simulink model "Stateflow_SD104"  (R2015b)
settings: Solver=FixedStepAuto  StartTime=0.0  StopTime=20  RelTol=1e-3
settings Model: Creator=amyyang  LastModifiedBy=amyyang
settings OptimizationCC: DefaultParameterBehavior=Inlined  OptimizeModelRefInitCode=on  LifeSpan=1
settings RTWCC: SystemTargetFile=ert.tlc  GenCodeOnly=on  TemplateMakefile=ert_default_tmf  Description=Embedded Coder  GenerateReport=on  IncludeHyperlinkInReport=on  LaunchReport=on  GenerateTraceInfo=on  GenerateTraceReport=on  GenerateTraceReportSl=on  GenerateTraceReportSf=on  GenerateTraceReportEml=on
settings CodeAppCC: IgnoreCustomStorageClasses=off
settings ERTTargetCC: GenerateSampleERTMain=on  InlinedParameterPlacement=NonHierarchical  ERTCustomFileTemplate=example_file_process.tlc

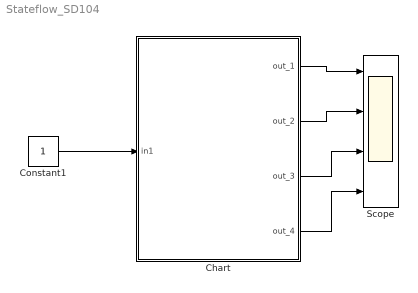
== system Stateflow_SD104 ==
  Chart : Stateflow chart  TreatAsAtomicUnit=on
  Constant1 : Constant
  Scope : Scope  NumInputPorts=4
  wires:
  Constant1/1 -> Chart/1(in1)
  Chart/1(out_1) -> Scope/1
  Chart/2(out_2) -> Scope/2
  Chart/3(out_3) -> Scope/3
  Chart/4(out_4) -> Scope/4

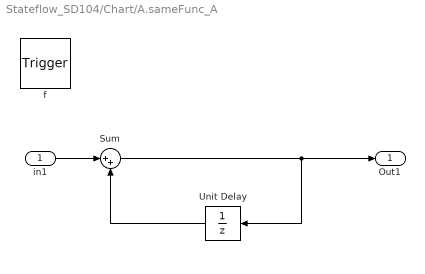
== system Stateflow_SD104/Chart/A.sameFunc_A ==
  in1 : Inport  OutDataTypeStr=double  PortDimensions=1
  f : TriggerPort  TriggerType=function-call
      settings: CopyFcn=Stateflow.SLINSF.SimulinkMan.removeBlockPreDeleteFcn  PreDeleteFcn=Stateflow.SLINSF.SimulinkMan.unsafePredeleteFcn
  Sum : Sum  Inputs=|++
  Unit Delay : UnitDelay  SampleTime=-1
  Out1 : Outport
  wires:
  in1/1 -> Sum/1
  Sum/1 -> Unit Delay/1, Out1/1
  Unit Delay/1 -> Sum/2

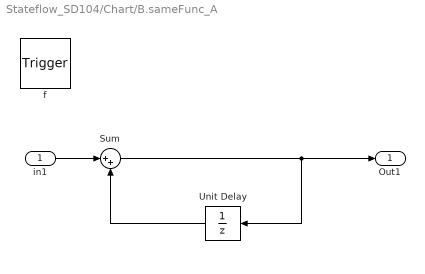
== system Stateflow_SD104/Chart/B.sameFunc_A ==
  in1 : Inport  OutDataTypeStr=double  PortDimensions=1
  f : TriggerPort  TriggerType=function-call
      settings: CopyFcn=Stateflow.SLINSF.SimulinkMan.removeBlockPreDeleteFcn  PreDeleteFcn=Stateflow.SLINSF.SimulinkMan.unsafePredeleteFcn
  Sum : Sum  Inputs=|++
  Unit Delay : UnitDelay  SampleTime=-1
  Out1 : Outport
  wires:
  in1/1 -> Sum/1
  Sum/1 -> Unit Delay/1, Out1/1
  Unit Delay/1 -> Sum/2

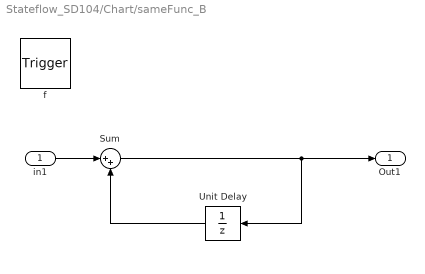
== system Stateflow_SD104/Chart/sameFunc_B ==
  in1 : Inport  OutDataTypeStr=double  PortDimensions=1
  f : TriggerPort  TriggerType=function-call
      settings: CopyFcn=Stateflow.SLINSF.SimulinkMan.removeBlockPreDeleteFcn  PreDeleteFcn=Stateflow.SLINSF.SimulinkMan.unsafePredeleteFcn
  Sum : Sum  Inputs=|++
  Unit Delay : UnitDelay  SampleTime=-1
  Out1 : Outport
  wires:
  in1/1 -> Sum/1
  Sum/1 -> Unit Delay/1, Out1/1
  Unit Delay/1 -> Sum/2

== stateflow chart Stateflow_SD104/Chart ==
  state A [parallel]
    du: out_1 = sameFunc_A(-2.0);
    settings: executionOrder=1
    state Out1 = sameFunc_A(in1) [function]
  state B [parallel]
    du: out_2 = sameFunc_A(2.0);
    settings: executionOrder=2
    state Out1 = sameFunc_A(in1) [function]
  state C [parallel]
    du: out_3 = sameFunc_B(-1.0);
    settings: executionOrder=3
  state D [parallel]
    du: out_4 = sameFunc_B(1.0);
    settings: executionOrder=4
  state Out1 = sameFunc_B(in1) [function]
  note: 图形函数基于父状态的可视范围
      | * 如果 在多个状态内 调用的函数是一样的， 单独有各自的状态 。如上。
      | *如果同一个函数被多次调用， 状态是共享的。如下。
      | 可以对比二者的 scope 的结果。
  note: Note: 在15b下，生成的代码函数都是重用的。
  data: in1 function_input double size=1; Out1 function_output; in1 function_input double size=1; Out1 function_output; in1 function_input double size=1; Out1 function_output; out_1 output; out_2 output; out_3 output; out_4 output; in1 input
